simulink model "ComputedTorque_iiwa"  (R2022b)
settings: Solver=ode4  StartTime=0.0  StopTime=T  FixedStep=0.001  RelTol=1e-3
values from neighbouring files (symbols this model uses):
  dq0 = ones(7,1)*pi/4    [init_ComputedTorque.m]    (also in init_ImpedanceController.m = zeros(7,1); init_PDplusController.m = zeros(7,1))
  k1 = kk    [init_ComputedTorque.m]
  k2 = kk    [init_ComputedTorque.m]
  q0 = [0; pi/4+0.5; 0; -pi/2; 0; pi/4+2;0]    [init_ComputedTorque.m]    (also in init_ImpedanceController.m = [0 pi/4 0 -pi/2 0 pi/4 0]'; init_PDplusController.m = [0 pi/4 0 -pi/2 0 pi/4 0]')
  T = 10    [init_ComputedTorque.m]    (also in init_ImpedanceController.m = 5; init_PDplusController.m = 5)
undefined symbols (not defined in the file or in its folder): param_robot, X, Y, Z
libraries: sm_lib x66, nesl_utility x8
(part 2 of 2)

== matlab function ComputedTorque_iiwa/RobotDynamics/MATLAB Function ==
  data: q input; ddq output; dq input; tau input
function ddq  = fcn(q,dq,tau)
    [M, C, g, ~, ~, ~] = dynamics_iiwa(q,dq);
    ddq = M\(-C*dq - g + tau);
end

== matlab function ComputedTorque_iiwa/MATLAB Function ==
  data: qd input; tau output; dqd input; ddqd input; q input; dq input; k1 input; k2 input
function tau = fcn(qd, dqd,ddqd, q, dq, k1, k2)

[M, C, g, ~, ~, ~] = dynamics_iiwa(q, dq);

K1 = eye(length(M))*k1;
K2 =eye(length(M))*k2;

tau = M*(ddqd-K2*(dq-dqd)- K1*(q-qd)) + C*dq +g;

== matlab function ComputedTorque_iiwa/JointSpace Trajectory/MATLAB Function2 ==
  data: t input; qd output; T input; dqd output; ddqd output
function [qd, dqd, ddqd] = fcn(t,T)
    Ttraj = 0.8*T;
    [qd, dqd, ddqd ]= jointspace_trajectory(t,Ttraj);
